simulink model "konvencionalni_PID"  (R2018a)
settings: Solver=ode4  StartTime=0.0  StopTime=100000.0  FixedStep=0.1  RelTol=1e-3
values from neighbouring files (symbols this model uses):
  Ca = 10^-6    (= 1e-06)    [projekat1.m]
  Cb = 10^-6    (= 1e-06)    [projekat1.m]
  Fa = 0.016667    [projekat1.m]
  K = 0.01    [projekat1.m]
  kw = 10^-14    (= 1e-14)    [projekat1.m]
  Ti = 65.1485    [projekat1.m]
  V = 30    [projekat1.m]
undefined symbols (not defined in the file or in its folder): Td, Tf
libraries: simulink x4
settings Model: Creator=svorc  LastModifiedBy=svorc
settings SolverCC: ZeroCrossAlgorithm=Adaptive
settings DataIOCC: ReturnWorkspaceOutputs=on
settings DebuggingCC: IgnoredZcDiagnostic=none  SFMachineParentedDataDiag=error
settings SFSimCC: SimUseLocalCustomCode=on
settings RTWCC: RTWUseLocalCustomCode=on

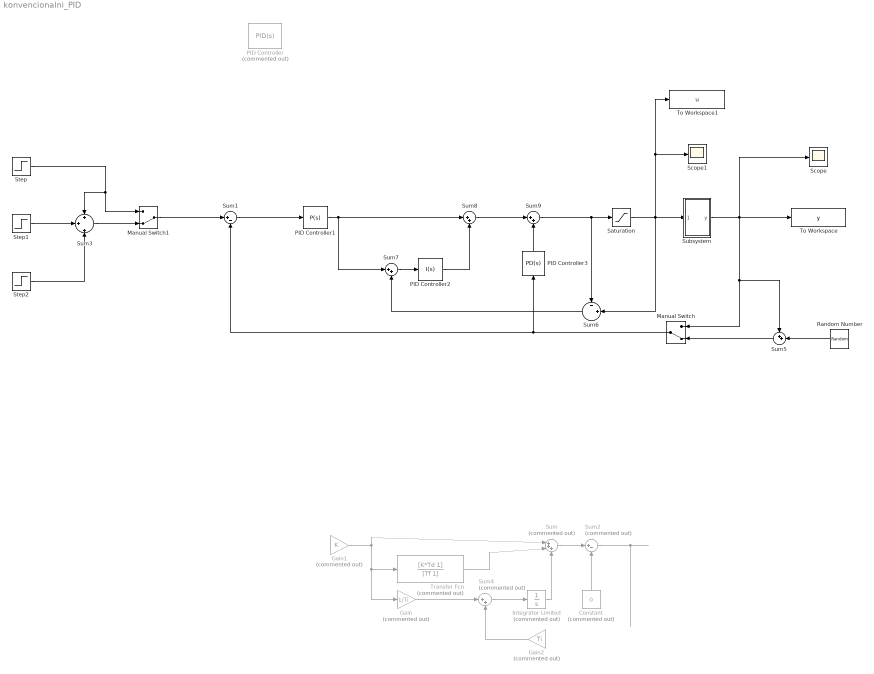
== system konvencionalni_PID ==
  Constant : Constant  Commented=on  Value=0
  Gain : Gain  Commented=on  Gain=1/Ti
  Gain1 : Gain  Commented=on  Gain=K
  Gain2 : Gain  Commented=on  Gain=Ti
  Integrator Limited : Integrator  Commented=on  LimitOutput=on  UpperSaturationLimit=10*Fa  LowerSaturationLimit=0
  Manual Switch : ManualSwitch  CurrentSetting=0
  Manual Switch1 : ManualSwitch  CurrentSetting=0
  PID Controller : simulink/Continuous/PID Controller  Commented=on  Controller=PID  Form=Parallel  TimeDomain=Continuous-time  SampleTime=-1  IntegratorMethod=Forward Euler  ControllerParametersSource=internal  P=K  I=1/Ti  D=Td  UseFilter=on  N=Tf  TunerSelectOption=Frequency Response Based  InitialConditionSource=internal  InitialConditionForIntegrator=0  InitialConditionForFilter=0  DifferentiatorICPrevScaledInput=0  ExternalReset=none  TrackingMode=off  Kt=1  LimitOutput=off  UpperSaturationLimit=inf  LowerSaturationLimit=-inf  LinearizeAsGain=on  AntiWindupMode=none  Kb=1  RndMeth=Round  POutMin=[]  POutMax=[]  IOutMin=[]  IOutMax=[]  DOutMin=[]  DOutMax=[]  NOutMin=[]  NOutMax=[]  SumOutMin=[]  SumOutMax=[]  SaturationOutMin=[]  SaturationOutMax=[]  PParamMin=[]  PParamMax=[]  IParamMin=[]  IParamMax=[]  DParamMin=[]  DParamMax=[]  NParamMin=[]  NParamMax=[]  KbParamMin=[]  KbParamMax=[]  KtParamMin=[]  KtParamMax=[]  KbOutMin=[]  KbOutMax=[]  KtOutMin=[]  KtOutMax=[]  IntegratorOutMin=[]  IntegratorOutMax=[]  FilterOutMin=[]  FilterOutMax=[]  SumI1OutMin=[]  SumI1OutMax=[]  SumI2OutMin=[]  SumI2OutMax=[]  SumI3OutMin=[]  SumI3OutMax=[]  SumDOutMin=[]  SumDOutMax=[]  DifferentiatorOutMin=[]  DifferentiatorOutMax=[]  FilterDiffOutCoefMin=[]  FilterDiffOutCoefMax=[]  ReciprocalOutMin=[]  ReciprocalOutMax=[]  SumDenOutMin=[]  SumDenOutMax=[]  SumNumOutMin=[]  SumNumOutMax=[]  DivideOutMin=[]  DivideOutMax=[]  IntegratorContinuousStateAttributes=''  IntegratorStateMustResolveToSignalObject=off  IntegratorRTWStateStorageClass=Auto  FilterContinuousStateAttributes=''  FilterStateMustResolveToSignalObject=off  FilterRTWStateStorageClass=Auto
  PID Controller1 : simulink/Continuous/PID Controller  Controller=P  Form=Parallel  TimeDomain=Continuous-time  SampleTime=-1  IntegratorMethod=Forward Euler  ControllerParametersSource=internal  P=K  I=1  D=0  UseFilter=on  N=100  TunerSelectOption=Transfer Function Based (PID Tuner App)  InitialConditionSource=internal  InitialConditionForIntegrator=0  InitialConditionForFilter=0  DifferentiatorICPrevScaledInput=0  ExternalReset=none  TrackingMode=off  Kt=1  LimitOutput=off  UpperSaturationLimit=inf  LowerSaturationLimit=-inf  LinearizeAsGain=on  AntiWindupMode=none  Kb=1  POutMin=[]  POutMax=[]  IOutMin=[]  IOutMax=[]  DOutMin=[]  DOutMax=[]  NOutMin=[]  NOutMax=[]  SumOutMin=[]  SumOutMax=[]  SaturationOutMin=[]  SaturationOutMax=[]  PParamMin=[]  PParamMax=[]  IParamMin=[]  IParamMax=[]  DParamMin=[]  DParamMax=[]  NParamMin=[]  NParamMax=[]  KbParamMin=[]  KbParamMax=[]  KtParamMin=[]  KtParamMax=[]  KbOutMin=[]  KbOutMax=[]  KtOutMin=[]  KtOutMax=[]  IntegratorOutMin=[]  IntegratorOutMax=[]  FilterOutMin=[]  FilterOutMax=[]  SumI1OutMin=[]  SumI1OutMax=[]  SumI2OutMin=[]  SumI2OutMax=[]  SumI3OutMin=[]  SumI3OutMax=[]  SumDOutMin=[]  SumDOutMax=[]  DifferentiatorOutMin=[]  DifferentiatorOutMax=[]  FilterDiffOutCoefMin=[]  FilterDiffOutCoefMax=[]  ReciprocalOutMin=[]  ReciprocalOutMax=[]  SumDenOutMin=[]  SumDenOutMax=[]  SumNumOutMin=[]  SumNumOutMax=[]  DivideOutMin=[]  DivideOutMax=[]  IntegratorContinuousStateAttributes=''  IntegratorStateMustResolveToSignalObject=off  IntegratorRTWStateStorageClass=Auto  FilterContinuousStateAttributes=''  FilterStateMustResolveToSignalObject=off  FilterRTWStateStorageClass=Auto
  PID Controller2 : simulink/Continuous/PID Controller  Controller=I  Form=Parallel  TimeDomain=Continuous-time  SampleTime=-1  IntegratorMethod=Forward Euler  ControllerParametersSource=internal  P=1  I=1/Ti  D=0  UseFilter=on  N=100  TunerSelectOption=Transfer Function Based (PID Tuner App)  InitialConditionSource=internal  InitialConditionForIntegrator=0  InitialConditionForFilter=0  DifferentiatorICPrevScaledInput=0  ExternalReset=none  TrackingMode=off  Kt=1  LimitOutput=off  UpperSaturationLimit=inf  LowerSaturationLimit=-inf  LinearizeAsGain=on  AntiWindupMode=none  Kb=1  POutMin=[]  POutMax=[]  IOutMin=[]  IOutMax=[]  DOutMin=[]  DOutMax=[]  NOutMin=[]  NOutMax=[]  SumOutMin=[]  SumOutMax=[]  SaturationOutMin=[]  SaturationOutMax=[]  PParamMin=[]  PParamMax=[]  IParamMin=[]  IParamMax=[]  DParamMin=[]  DParamMax=[]  NParamMin=[]  NParamMax=[]  KbParamMin=[]  KbParamMax=[]  KtParamMin=[]  KtParamMax=[]  KbOutMin=[]  KbOutMax=[]  KtOutMin=[]  KtOutMax=[]  IntegratorOutMin=[]  IntegratorOutMax=[]  FilterOutMin=[]  FilterOutMax=[]  SumI1OutMin=[]  SumI1OutMax=[]  SumI2OutMin=[]  SumI2OutMax=[]  SumI3OutMin=[]  SumI3OutMax=[]  SumDOutMin=[]  SumDOutMax=[]  DifferentiatorOutMin=[]  DifferentiatorOutMax=[]  FilterDiffOutCoefMin=[]  FilterDiffOutCoefMax=[]  ReciprocalOutMin=[]  ReciprocalOutMax=[]  SumDenOutMin=[]  SumDenOutMax=[]  SumNumOutMin=[]  SumNumOutMax=[]  DivideOutMin=[]  DivideOutMax=[]  IntegratorContinuousStateAttributes=''  IntegratorStateMustResolveToSignalObject=off  IntegratorRTWStateStorageClass=Auto  FilterContinuousStateAttributes=''  FilterStateMustResolveToSignalObject=off  FilterRTWStateStorageClass=Auto
  PID Controller3 : simulink/Continuous/PID Controller  Controller=PD  Form=Ideal  TimeDomain=Continuous-time  SampleTime=-1  IntegratorMethod=Forward Euler  ControllerParametersSource=internal  P=K  I=1  D=1/Td  UseFilter=on  N=Tf  TunerSelectOption=Transfer Function Based (PID Tuner App)  InitialConditionSource=internal  InitialConditionForIntegrator=0  InitialConditionForFilter=0  DifferentiatorICPrevScaledInput=0  ExternalReset=none  TrackingMode=off  Kt=1  LimitOutput=off  UpperSaturationLimit=inf  LowerSaturationLimit=-inf  LinearizeAsGain=on  AntiWindupMode=none  Kb=1  POutMin=[]  POutMax=[]  IOutMin=[]  IOutMax=[]  DOutMin=[]  DOutMax=[]  NOutMin=[]  NOutMax=[]  SumOutMin=[]  SumOutMax=[]  SaturationOutMin=[]  SaturationOutMax=[]  PParamMin=[]  PParamMax=[]  IParamMin=[]  IParamMax=[]  DParamMin=[]  DParamMax=[]  NParamMin=[]  NParamMax=[]  KbParamMin=[]  KbParamMax=[]  KtParamMin=[]  KtParamMax=[]  KbOutMin=[]  KbOutMax=[]  KtOutMin=[]  KtOutMax=[]  IntegratorOutMin=[]  IntegratorOutMax=[]  FilterOutMin=[]  FilterOutMax=[]  SumI1OutMin=[]  SumI1OutMax=[]  SumI2OutMin=[]  SumI2OutMax=[]  SumI3OutMin=[]  SumI3OutMax=[]  SumDOutMin=[]  SumDOutMax=[]  DifferentiatorOutMin=[]  DifferentiatorOutMax=[]  FilterDiffOutCoefMin=[]  FilterDiffOutCoefMax=[]  ReciprocalOutMin=[]  ReciprocalOutMax=[]  SumDenOutMin=[]  SumDenOutMax=[]  SumNumOutMin=[]  SumNumOutMax=[]  DivideOutMin=[]  DivideOutMax=[]  IntegratorContinuousStateAttributes=''  IntegratorStateMustResolveToSignalObject=off  IntegratorRTWStateStorageClass=Auto  FilterContinuousStateAttributes=''  FilterStateMustResolveToSignalObject=off  FilterRTWStateStorageClass=Auto
  Random Number : RandomNumber  Variance=0.01225  SampleTime=0.1
  Saturation : Saturate  UpperLimit=10*Fa  LowerLimit=0
  Scope : Scope
  Scope1 : Scope
  Step : Step  Time=0.1  After=7  SampleTime=0
  Step1 : Step  Time=10000  After=-0.8  SampleTime=0
  Step2 : Step  Time=50000  After=1.3  SampleTime=0
  Subsystem : Subsystem
  Sum : Sum  Commented=on  Inputs=|+++
  Sum1 : Sum  Inputs=|+-
  Sum2 : Sum  Commented=on  Inputs=|+-
  Sum3 : Sum  Inputs=+|+|+
  Sum4 : Sum  Commented=on  Inputs=|++
  Sum5 : Sum  Inputs=++|
  Sum6 : Sum  Inputs=-|+||
  Sum7 : Sum  Inputs=|++
  Sum8 : Sum  Inputs=|++
  Sum9 : Sum  Inputs=|++
  To Workspace : ToWorkspace  VariableName=y  SampleTime=-1
  To Workspace1 : ToWorkspace  VariableName=u  SampleTime=-1
  Transfer Fcn : TransferFcn  Commented=on  Numerator=[K*Td 1]  Denominator=[Tf 1]
  wires:
  Saturation/1 -> Sum6/2, To Workspace1/1, Scope1/1, Subsystem/1(Input)
  Sum3/1 -> Manual Switch1/2
  Manual Switch1/1 -> Sum1/1
  Step2/1 -> Sum3/3
  Step/1 -> Manual Switch1/1, Sum3/1
  Step1/1 -> Sum3/2
  Random Number/1 -> Sum5/2
  Sum5/1 -> Manual Switch/2
  Subsystem/1(y) -> Manual Switch/1, Sum5/1, To Workspace/1, Scope/1
  Manual Switch/1 -> PID Controller3/1, Sum1/2
  Integrator Limited/1 -> Sum/3
  Sum4/1 -> Integrator Limited/1
  Gain/1 -> Sum4/1
  Gain2/1 -> Sum4/2
  ? -> Gain1/1
  Sum/1 -> Sum2/1
  ? -> Gain2/1
  Transfer Fcn/1 -> Sum/2
  Sum2/1 -> ?
  Constant/1 -> Sum2/2
  Gain1/1 -> Sum/1, Gain/1, Transfer Fcn/1
  Sum1/1 -> PID Controller1/1
  Sum8/1 -> Sum9/1
  Sum9/1 -> Sum6/1, Saturation/1
  PID Controller3/1 -> Sum9/2
  Sum6/1 -> Sum7/2
  PID Controller1/1 -> Sum7/1, Sum8/1
  Sum7/1 -> PID Controller2/1
  PID Controller2/1 -> Sum8/2

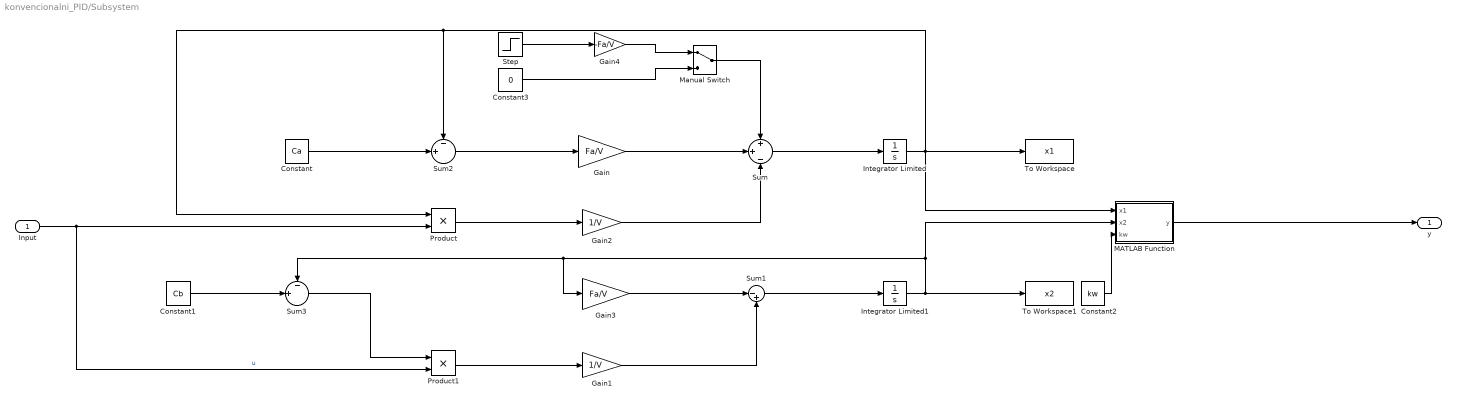
== system konvencionalni_PID/Subsystem ==
  Input : Inport
  Constant : Constant  Value=Ca
  Constant1 : Constant  Value=Cb
  Constant2 : Constant  Value=kw
  Constant3 : Constant  Value=0
  Gain : Gain  Gain=Fa/V
  Gain1 : Gain  Gain=1/V
  Gain2 : Gain  Gain=1/V
  Gain3 : Gain  Gain=Fa/V
  Gain4 : Gain  Gain=-Fa/V
  Integrator Limited : Integrator  LimitOutput=on  UpperSaturationLimit=Ca  LowerSaturationLimit=0
  Integrator Limited1 : Integrator  LimitOutput=on  UpperSaturationLimit=Cb  LowerSaturationLimit=0
  MATLAB Function : MATLAB Function  TreatAsAtomicUnit=on
  Manual Switch : ManualSwitch
  Product : Product
  Product1 : Product
  Step : Step  Time=70000  After=Ca  SampleTime=0
  Sum : Sum  Inputs=+|+|-
  Sum1 : Sum  Inputs=|-+
  Sum2 : Sum  Inputs=-|+||
  Sum3 : Sum  Inputs=-|+||
  To Workspace : ToWorkspace  VariableName=x1  SampleTime=-1
  To Workspace1 : ToWorkspace  VariableName=x2  SampleTime=-1
  y : Outport
  wires:
  Sum3/1 -> Product1/1
  Sum/1 -> Integrator Limited/1
  Input/1 -> Product/2, Product1/2  "u"
  Gain3/1 -> Sum1/1
  Integrator Limited1/1 -> MATLAB Function/2(x2), Gain3/1, Sum3/1, To Workspace1/1
  Integrator Limited/1 -> To Workspace/1, MATLAB Function/1(x1), Sum2/1, Product/1
  Constant1/1 -> Sum3/2
  Sum1/1 -> Integrator Limited1/1
  Product1/1 -> Gain1/1
  Constant/1 -> Sum2/2
  MATLAB Function/1(y) -> y/1
  Gain1/1 -> Sum1/2
  Product/1 -> Gain2/1
  Sum2/1 -> Gain/1
  Constant2/1 -> MATLAB Function/3(kw)
  Gain2/1 -> Sum/3
  Gain/1 -> Sum/2
  Manual Switch/1 -> Sum/1
  Gain4/1 -> Manual Switch/1
  Step/1 -> Gain4/1
  Constant3/1 -> Manual Switch/2

== matlab function konvencionalni_PID/Subsystem/MATLAB Function ==
  data: x1 input; y output; x2 input; kw input
function y = fcn(x1, x2, kw)

y = -log10(sqrt((x2-x1)^2 / 4 + kw) - (x2 - x1) / 2);
